simulink model "VehCtrl20260630_18B"  (R2018b)
settings: Solver=FixedStepAuto  StartTime=0.0  StopTime=inf  FixedStep=0.005  RelTol=1e-3
InitFcn:
  | mbd_mpc_consistency_checks(bdroot(gcs));
undefined symbols (not defined in the file): ANG_DEAD, BMS_NormalPwr, BrakeDeadZone, BrkPrsByBrkPct_TB_X, BrkPrsByBrkPct_TB_Y, DELAY_DISCHARGE, DELAY_RCUOFF, DRV_BACKWARD, DRV_BRAKE, DRV_FORWARD, DRV_NEUTRAL, DRV_PARK, DRV_UNPARK, DRV_ZEROTURN, EPB_LOCK, EPB_UNLOCK, ExtraLoadPwr, FanOff, fifo_0_vect, fifo_1_vect, HiFanReq, HV_finished, HV_No_Active, HV_POWER_OFF, HV_POWER_ON, HVDown, HVON, KaTLS_v_DrgUp_X_VehSpd, KeFTM_s_Way1OffDlyTime, KeFTM_TK_Way1CoolLv2OffBatTemp, KeFTM_TK_Way1CoolLv2OffMtrTemp, KeFTM_TK_Way1CoolLv2OnBatTemp, KeFTM_TK_Way1CoolLv2OnMtrTemp, KeFTM_TK_Way1CoolLv3OffBatTemp, KeFTM_TK_Way1CoolLv3OffMtrTemp, KeFTM_TK_Way1CoolLv3OnBatTemp, KeFTM_TK_Way1CoolLv3OnMtrTemp, KeFTM_TK_Way1CoolLv4OffBatTemp, KeFTM_TK_Way1CoolLv4OffMtrTemp, KeFTM_TK_Way1CoolLv4OnBatTemp, KeFTM_TK_Way1CoolLv4OnMtrTemp, Kp1, Kp2, LowFanReq, LQFP, MtrCmdGainFL, MtrCmdGainFR, MtrCmdGainRL, MtrCmdGainRR, MtrPwrFactor_RCU, MtrPwrHighToMidThd, MtrPwrLowToMidThd, MtrPwrMidToHighThd, MtrPwrMidToLowThd, MtrTrqMax, PCT_DEAD, Precharge, PTO_1000, PTO_540, pts1_fifo_0_vect ... (+32)
libraries: mbd_mpc574x_ec_toolbox x175, simulink x110, canmsglib x70
(part 3 of 15)

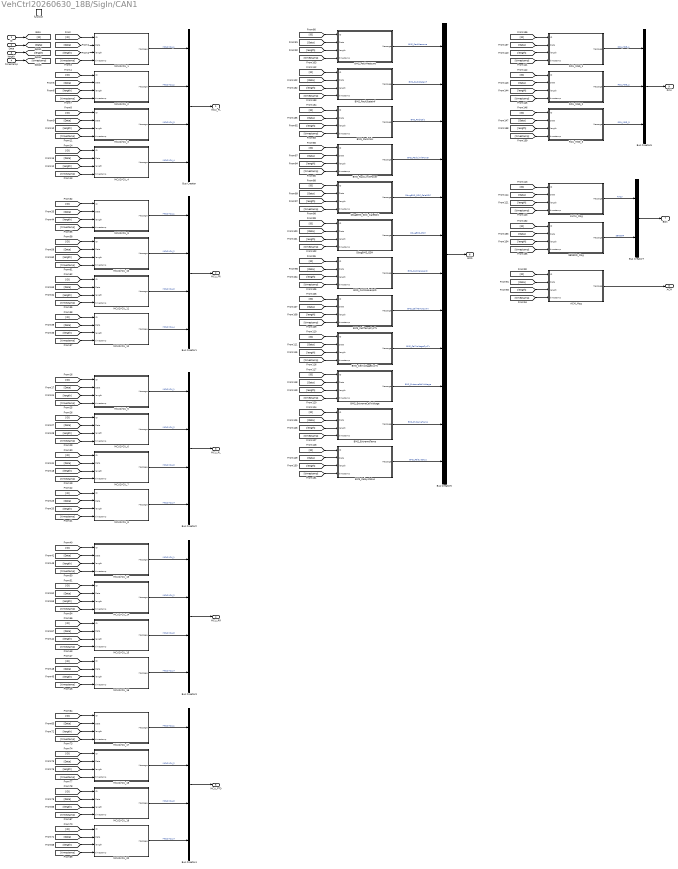
== system VehCtrl20260630_18B/SigIn/CAN1 ==
  ID : Inport
  Data : Inport  Port=2
  length : Inport  Port=3
  timestamp : Inport  Port=4
  function : TriggerPort  TriggerType=function-call  VariantControl=Variant
  ACM_Msg : Subsystem
  AVCU_Msg : Subsystem
  BMS_CANWakeUpID : Subsystem
  BMS_CellTempCycTx : Subsystem
  BMS_CellVoltageCycTx : Subsystem
  BMS_ExtremeCellVoltage : Subsystem
  BMS_ExtremeTemp : Subsystem
  BMS_PackCalc : Subsystem
  BMS_PackLimitPower : Subsystem
  BMS_PackMeasure : Subsystem
  BMS_PackStateInf : Subsystem
  BMS_Relaystatus : Subsystem
  Bus Creator{,1..4} (5 alike) : BusCreator  Inputs=4
  Bus Creator5 : BusCreator  Inputs=12
  Bus Creator6 : BusCreator  Inputs=3
  Bus Creator7 : BusCreator  Inputs=2
  DbugBMS_ESM : Subsystem
  DbugBMS_SOC_CaleSOC : Subsystem
  MCU2VCU_1 : Subsystem
  MCU2VCU_10 : Subsystem
  MCU2VCU_11 : Subsystem
  MCU2VCU_12 : Subsystem
  MCU2VCU_13 : Subsystem
  MCU2VCU_14 : Subsystem
  MCU2VCU_15 : Subsystem
  MCU2VCU_16 : Subsystem
  MCU2VCU_17 : Subsystem
  MCU2VCU_18 : Subsystem
  MCU2VCU_19 : Subsystem
  MCU2VCU_2 : Subsystem
  MCU2VCU_20 : Subsystem
  MCU2VCU_3 : Subsystem
  MCU2VCU_4 : Subsystem
  MCU2VCU_5 : Subsystem
  MCU2VCU_6 : Subsystem
  MCU2VCU_7 : Subsystem
  MCU2VCU_8 : Subsystem
  MCU2VCU_9 : Subsystem
  RCU_MSG_1 : Subsystem
  RCU_MSG_2 : Subsystem
  RCU_MSG_3 : Subsystem
  SENSOR_Msg : Subsystem
  MCU_FL : Outport
  MCU_FR : Outport  Port=2
  MCU_RL : Outport  Port=3
  MCU_RR : Outport  Port=4
  MCU_PTO : Outport  Port=5
  BMS : Outport  Port=6
  BDX : Outport  Port=7
  ACM : Outport  Port=8
  RCU : Outport  Port=9
  wires:
  Bus Creator/1 -> MCU_FL/1
  ID/1 -> [ID]
  Data/1 -> [Data]
  timestamp/1 -> [timestamp]
  length/1 -> [length]
  [ID] -> MCU2VCU_1/1(ID)
  [Data] -> MCU2VCU_1/2(Data)
  [length] -> MCU2VCU_1/3(length)
  [timestamp] -> MCU2VCU_1/4(timestamp)
  [timestamp] -> MCU2VCU_2/4(timestamp)
  [length] -> MCU2VCU_2/3(length)
  [Data] -> MCU2VCU_2/2(Data)
  [ID] -> MCU2VCU_2/1(ID)
  [ID] -> MCU2VCU_3/1(ID)
  [Data] -> MCU2VCU_3/2(Data)
  [length] -> MCU2VCU_3/3(length)
  [timestamp] -> MCU2VCU_3/4(timestamp)
  [timestamp] -> MCU2VCU_4/4(timestamp)
  [length] -> MCU2VCU_4/3(length)
  [Data] -> MCU2VCU_4/2(Data)
  [ID] -> MCU2VCU_4/1(ID)
  MCU2VCU_1/1(Message) -> Bus Creator/1  "MCU2VCU_1"
  MCU2VCU_2/1(Message) -> Bus Creator/2  "MCU2VCU_2"
  MCU2VCU_3/1(Message) -> Bus Creator/3  "MCU2VCU_3"
  MCU2VCU_4/1(Message) -> Bus Creator/4  "MCU2VCU_4"
  MCU2VCU_8/1(Message) -> Bus Creator2/4  "MCU2VCU_4"
  MCU2VCU_7/1(Message) -> Bus Creator2/3  "MCU2VCU_3"
  MCU2VCU_6/1(Message) -> Bus Creator2/2  "MCU2VCU_2"
  MCU2VCU_5/1(Message) -> Bus Creator2/1  "MCU2VCU_1"
  [ID] -> MCU2VCU_8/1(ID)
  [Data] -> MCU2VCU_8/2(Data)
  [length] -> MCU2VCU_8/3(length)
  [timestamp] -> MCU2VCU_8/4(timestamp)
  [timestamp] -> MCU2VCU_7/4(timestamp)
  [length] -> MCU2VCU_7/3(length)
  [Data] -> MCU2VCU_7/2(Data)
  [ID] -> MCU2VCU_7/1(ID)
  [ID] -> MCU2VCU_6/1(ID)
  [Data] -> MCU2VCU_6/2(Data)
  [length] -> MCU2VCU_6/3(length)
  [timestamp] -> MCU2VCU_6/4(timestamp)
  [timestamp] -> MCU2VCU_5/4(timestamp)
  [length] -> MCU2VCU_5/3(length)
  [Data] -> MCU2VCU_5/2(Data)
  [ID] -> MCU2VCU_5/1(ID)
  Bus Creator2/1 -> MCU_RL/1
  Bus Creator3/1 -> MCU_RR/1
  [ID] -> MCU2VCU_13/1(ID)
  [Data] -> MCU2VCU_13/2(Data)
  [length] -> MCU2VCU_13/3(length)
  [timestamp] -> MCU2VCU_13/4(timestamp)
  [timestamp] -> MCU2VCU_14/4(timestamp)
  [length] -> MCU2VCU_14/3(length)
  [Data] -> MCU2VCU_14/2(Data)
  [ID] -> MCU2VCU_14/1(ID)
  [ID] -> MCU2VCU_15/1(ID)
  [Data] -> MCU2VCU_15/2(Data)
  [length] -> MCU2VCU_15/3(length)
  [timestamp] -> MCU2VCU_15/4(timestamp)
  [timestamp] -> MCU2VCU_16/4(timestamp)
  [length] -> MCU2VCU_16/3(length)
  [Data] -> MCU2VCU_16/2(Data)
  [ID] -> MCU2VCU_16/1(ID)
  MCU2VCU_13/1(Message) -> Bus Creator3/1  "MCU2VCU_1"
  MCU2VCU_14/1(Message) -> Bus Creator3/2  "MCU2VCU_2"
  MCU2VCU_15/1(Message) -> Bus Creator3/3  "MCU2VCU_3"
  MCU2VCU_16/1(Message) -> Bus Creator3/4  "MCU2VCU_4"
  MCU2VCU_12/1(Message) -> Bus Creator1/4  "MCU2VCU_4"
  MCU2VCU_11/1(Message) -> Bus Creator1/3  "MCU2VCU_3"
  MCU2VCU_10/1(Message) -> Bus Creator1/2  "MCU2VCU_2"
  MCU2VCU_9/1(Message) -> Bus Creator1/1  "MCU2VCU_1"
  [ID] -> MCU2VCU_12/1(ID)
  [Data] -> MCU2VCU_12/2(Data)
  [length] -> MCU2VCU_12/3(length)
  [timestamp] -> MCU2VCU_12/4(timestamp)
  [timestamp] -> MCU2VCU_11/4(timestamp)
  [length] -> MCU2VCU_11/3(length)
  [Data] -> MCU2VCU_11/2(Data)
  [ID] -> MCU2VCU_11/1(ID)
  [ID] -> MCU2VCU_10/1(ID)
  [Data] -> MCU2VCU_10/2(Data)
  [length] -> MCU2VCU_10/3(length)
  [timestamp] -> MCU2VCU_10/4(timestamp)
  [timestamp] -> MCU2VCU_9/4(timestamp)
  [length] -> MCU2VCU_9/3(length)
  [Data] -> MCU2VCU_9/2(Data)
  [ID] -> MCU2VCU_9/1(ID)
  Bus Creator1/1 -> MCU_FR/1
  MCU2VCU_20/1(Message) -> Bus Creator4/4  "MCU2VCU_4"
  MCU2VCU_19/1(Message) -> Bus Creator4/3  "MCU2VCU_3"
  MCU2VCU_18/1(Message) -> Bus Creator4/2  "MCU2VCU_2"
  MCU2VCU_17/1(Message) -> Bus Creator4/1  "MCU2VCU_1"
  [ID] -> MCU2VCU_20/1(ID)
  [Data] -> MCU2VCU_20/2(Data)
  [length] -> MCU2VCU_20/3(length)
  [timestamp] -> MCU2VCU_20/4(timestamp)
  [timestamp] -> MCU2VCU_19/4(timestamp)
  [length] -> MCU2VCU_19/3(length)
  [Data] -> MCU2VCU_19/2(Data)
  [ID] -> MCU2VCU_19/1(ID)
  [ID] -> MCU2VCU_18/1(ID)
  [Data] -> MCU2VCU_18/2(Data)
  [length] -> MCU2VCU_18/3(length)
  [timestamp] -> MCU2VCU_18/4(timestamp)
  [timestamp] -> MCU2VCU_17/4(timestamp)
  [length] -> MCU2VCU_17/3(length)
  [Data] -> MCU2VCU_17/2(Data)
  [ID] -> MCU2VCU_17/1(ID)
  Bus Creator4/1 -> MCU_PTO/1
  [timestamp] -> BMS_CellTempCycTx/4(timestamp)
  [timestamp] -> ACM_Msg/4(timestamp)
  [ID] -> BMS_Relaystatus/1(ID)
  BMS_ExtremeCellVoltage/1(Message) -> Bus Creator5/10  "BMS_ExtremeCellVoltage"
  [Data] -> DbugBMS_ESM/2(Data)
  BMS_CellTempCycTx/1(Message) -> Bus Creator5/8  "BMS_CellTempCycTx"
  BMS_CellVoltageCycTx/1(Message) -> Bus Creator5/9  "BMS_CellVoltageCycTx"
  [ID] -> AVCU_Msg/1(ID)
  [length] -> BMS_Relaystatus/3(length)
  [timestamp] -> BMS_CANWakeUpID/4(timestamp)
  [length] -> BMS_CellTempCycTx/3(length)
  DbugBMS_SOC_CaleSOC/1(Message) -> Bus Creator5/5  "DbugBMS_SOC_CaleSOC"
  [timestamp] -> BMS_Relaystatus/4(timestamp)
  [timestamp] -> BMS_PackStateInf/4(timestamp)
  [ID] -> BMS_ExtremeCellVoltage/1(ID)
  BMS_Relaystatus/1(Message) -> Bus Creator5/12  "BMS_Relaystatus"
  [Data] -> BMS_CANWakeUpID/2(Data)
  [length] -> BMS_ExtremeCellVoltage/3(length)
  [timestamp] -> BMS_ExtremeCellVoltage/4(timestamp)
  [Data] -> BMS_PackLimitPower/2(Data)
  [Data] -> BMS_ExtremeCellVoltage/2(Data)
  [Data] -> BMS_PackStateInf/2(Data)
  [Data] -> BMS_ExtremeTemp/2(Data)
  DbugBMS_ESM/1(Message) -> Bus Creator5/6  "DbugBMS_ESM"
  [timestamp] -> BMS_PackCalc/4(timestamp)
  [ID] -> BMS_CANWakeUpID/1(ID)
  [Data] -> BMS_CellTempCycTx/2(Data)
  [length] -> AVCU_Msg/3(length)
  [length] -> BMS_PackCalc/3(length)
  [ID] -> ACM_Msg/1(ID)
  [timestamp] -> BMS_CellVoltageCycTx/4(timestamp)
  ACM_Msg/1(Message) -> ACM/1
  Bus Creator5/1 -> BMS/1
  [length] -> ACM_Msg/3(length)
  [Data] -> BMS_PackMeasure/2(Data)
  [timestamp] -> BMS_PackLimitPower/4(timestamp)
  [Data] -> BMS_CellVoltageCycTx/2(Data)
  [ID] -> BMS_PackLimitPower/1(ID)
  [Data] -> DbugBMS_SOC_CaleSOC/2(Data)
  BMS_CANWakeUpID/1(Message) -> Bus Creator5/7  "BMS_CANWakeUpID"
  [ID] -> BMS_PackCalc/1(ID)
  [length] -> BMS_PackMeasure/3(length)
  BMS_PackMeasure/1(Message) -> Bus Creator5/1  "BMS_PackMeasure"
  [Data] -> BMS_Relaystatus/2(Data)
  [Data] -> BMS_PackCalc/2(Data)
  [length] -> BMS_PackLimitPower/3(length)
  [ID] -> BMS_ExtremeTemp/1(ID)
  BMS_PackCalc/1(Message) -> Bus Creator5/3  "BMS_PackCalc"
  [timestamp] -> BMS_ExtremeTemp/4(timestamp)
  BMS_PackStateInf/1(Message) -> Bus Creator5/2  "BMS_PackStateInf"
  [length] -> BMS_CellVoltageCycTx/3(length)
  [timestamp] -> DbugBMS_ESM/4(timestamp)
  [ID] -> BMS_CellVoltageCycTx/1(ID)
  [length] -> BMS_CANWakeUpID/3(length)
  [length] -> DbugBMS_ESM/3(length)
  BMS_PackLimitPower/1(Message) -> Bus Creator5/4  "BMS_PackLimitPower"
  [ID] -> DbugBMS_SOC_CaleSOC/1(ID)
  [length] -> BMS_ExtremeTemp/3(length)
  [timestamp] -> DbugBMS_SOC_CaleSOC/4(timestamp)
  [ID] -> BMS_PackStateInf/1(ID)
  [Data] -> ACM_Msg/2(Data)
  [ID] -> BMS_CellTempCycTx/1(ID)
  [Data] -> AVCU_Msg/2(Data)
  [ID] -> BMS_PackMeasure/1(ID)
  [timestamp] -> BMS_PackMeasure/4(timestamp)
  BMS_ExtremeTemp/1(Message) -> Bus Creator5/11  "BMS_ExtremeTemp"
  [ID] -> DbugBMS_ESM/1(ID)
  [length] -> BMS_PackStateInf/3(length)
  [timestamp] -> AVCU_Msg/4(timestamp)
  [length] -> DbugBMS_SOC_CaleSOC/3(length)
  RCU_MSG_2/1(Message) -> Bus Creator6/2  "RCU_MSG_2"
  [length] -> RCU_MSG_3/3(length)
  RCU_MSG_3/1(Message) -> Bus Creator6/3  "RCU_MSG_3"
  [Data] -> RCU_MSG_2/2(Data)
  [length] -> RCU_MSG_2/3(length)
  [Data] -> RCU_MSG_1/2(Data)
  [Data] -> RCU_MSG_3/2(Data)
  [ID] -> RCU_MSG_2/1(ID)
  [timestamp] -> RCU_MSG_2/4(timestamp)
  [ID] -> RCU_MSG_3/1(ID)
  RCU_MSG_1/1(Message) -> Bus Creator6/1  "RCU_MSG_1"
  [length] -> RCU_MSG_1/3(length)
  [ID] -> RCU_MSG_1/1(ID)
  [timestamp] -> RCU_MSG_3/4(timestamp)
  Bus Creator6/1 -> RCU/1
  [timestamp] -> RCU_MSG_1/4(timestamp)
  [ID] -> SENSOR_Msg/1(ID)
  [Data] -> SENSOR_Msg/2(Data)
  [length] -> SENSOR_Msg/3(length)
  [timestamp] -> SENSOR_Msg/4(timestamp)
  SENSOR_Msg/1(Message) -> Bus Creator7/2  "SENSOR"
  AVCU_Msg/1(Message) -> Bus Creator7/1  "AVCU"
  Bus Creator7/1 -> BDX/1

== system VehCtrl20260630_18B/SigIn/DI ==
  note: DI PULLDOWN
  note: DI PULLUP
  Bus Creator : BusCreator  Inputs=14
  DI01 : mbd_mpc574x_ec_toolbox/GPIO Blocks/Digital_Input  gpio_pin=PTG5: [SIUL2_GPIO101 | General Purpose IO PG[5]]  pull_resistor=None
  DI02 : mbd_mpc574x_ec_toolbox/GPIO Blocks/Digital_Input  gpio_pin=PTG9: [SIUL2_GPIO105 | General Purpose IO PG[9]]  pull_resistor=None
  DI03 : mbd_mpc574x_ec_toolbox/GPIO Blocks/Digital_Input  gpio_pin=PTC11: [SIUL2_GPIO43 | General Purpose IO PC[11]]  pull_resistor=None
  DI04 : mbd_mpc574x_ec_toolbox/GPIO Blocks/Digital_Input  gpio_pin=PTA9: [SIUL2_GPIO9 | General Purpose IO PA[9]]  pull_resistor=None
  DI07 : mbd_mpc574x_ec_toolbox/GPIO Blocks/Digital_Input  gpio_pin=PTA0: [SIUL2_GPIO0 | General Purpose IO PA[0]]  pull_resistor=None
  DI08 : mbd_mpc574x_ec_toolbox/GPIO Blocks/Digital_Input  gpio_pin=PTD11: [SIUL2_GPIO59 | General Purpose IO PD[11]]  pull_resistor=None
  DI09 : mbd_mpc574x_ec_toolbox/GPIO Blocks/Digital_Input  gpio_pin=PTG6: [SIUL2_GPIO102 | General Purpose IO PG[6]]  pull_resistor=None
  DI10 : mbd_mpc574x_ec_toolbox/GPIO Blocks/Digital_Input  gpio_pin=PTG2: [SIUL2_GPIO98 | General Purpose IO PG[2]]  pull_resistor=None
  DI12 : mbd_mpc574x_ec_toolbox/GPIO Blocks/Digital_Input  gpio_pin=PTF13: [SIUL2_GPIO93 | General Purpose IO PF[13]]  pull_resistor=None
  DI13 : mbd_mpc574x_ec_toolbox/GPIO Blocks/Digital_Input  gpio_pin=PTG4: [SIUL2_GPIO100 | General Purpose IO PG[4]]  pull_resistor=None
  DI15 : mbd_mpc574x_ec_toolbox/GPIO Blocks/Digital_Input  gpio_pin=PTF12: [SIUL2_GPIO92 | General Purpose IO PF[12]]  pull_resistor=None
  DI16 : mbd_mpc574x_ec_toolbox/GPIO Blocks/Digital_Input  gpio_pin=PTG7: [SIUL2_GPIO103 | General Purpose IO PG[7]]  pull_resistor=None
  DI17 : mbd_mpc574x_ec_toolbox/GPIO Blocks/Digital_Input  gpio_pin=PTD10: [SIUL2_GPIO58 | General Purpose IO PD[10]]  pull_resistor=None
  DI18 : mbd_mpc574x_ec_toolbox/GPIO Blocks/Digital_Input  gpio_pin=PTG10: [SIUL2_GPIO106 | General Purpose IO PG[10]]  pull_resistor=None
  DI_31_32_33_34 : Subsystem  Commented=on
  Data Store Read : DataStoreRead  DataStoreName=DI07
  Data Store Read1 : DataStoreRead  DataStoreName=DI10
  Data Store Read10 : DataStoreRead  DataStoreName=DI04
  Data Store Read11 : DataStoreRead  DataStoreName=DI12
  Data Store Read12 : DataStoreRead  DataStoreName=DI08
  Data Store Read13 : DataStoreRead  DataStoreName=DI09
  Data Store Read2 : DataStoreRead  DataStoreName=DI13
  Data Store Read3 : DataStoreRead  DataStoreName=DI15
  Data Store Read4 : DataStoreRead  DataStoreName=DI16
  Data Store Read5 : DataStoreRead  DataStoreName=DI17
  Data Store Read6 : DataStoreRead  DataStoreName=DI18
  Data Store Read7 : DataStoreRead  DataStoreName=DI01
  Data Store Read8 : DataStoreRead  DataStoreName=DI02
  Data Store Read9 : DataStoreRead  DataStoreName=DI03
  Data Store Write : DataStoreWrite  DataStoreName=DI07
  Data Store Write1 : DataStoreWrite  DataStoreName=DI01
  Data Store Write10 : DataStoreWrite  DataStoreName=DI04
  Data Store Write11 : DataStoreWrite  DataStoreName=DI12
  Data Store Write12 : DataStoreWrite  DataStoreName=DI08
  Data Store Write13 : DataStoreWrite  DataStoreName=DI09
  Data Store Write2 : DataStoreWrite  DataStoreName=DI10
  Data Store Write3 : DataStoreWrite  DataStoreName=DI13
  Data Store Write4 : DataStoreWrite  DataStoreName=DI15
  Data Store Write5 : DataStoreWrite  DataStoreName=DI16
  Data Store Write6 : DataStoreWrite  DataStoreName=DI17
  Data Store Write7 : DataStoreWrite  DataStoreName=DI18
  Data Store Write8 : DataStoreWrite  DataStoreName=DI02
  Data Store Write9 : DataStoreWrite  DataStoreName=DI03
  DI : Outport
  wires:
  DI07/1 -> Data Store Write/1
  DI01/1 -> Data Store Write1/1
  DI10/1 -> Data Store Write2/1
  DI13/1 -> Data Store Write3/1
  DI15/1 -> Data Store Write4/1
  DI17/1 -> Data Store Write6/1
  DI16/1 -> Data Store Write5/1
  DI18/1 -> Data Store Write7/1
  DI09/1 -> Data Store Write13/1
  DI08/1 -> Data Store Write12/1
  DI12/1 -> Data Store Write11/1
  DI04/1 -> Data Store Write10/1
  DI02/1 -> Data Store Write8/1
  DI03/1 -> Data Store Write9/1
  Data Store Read/1 -> Bus Creator/1  "DI07"
  Data Store Read1/1 -> Bus Creator/2  "DI10"
  Data Store Read2/1 -> Bus Creator/3  "DI13"
  Data Store Read3/1 -> Bus Creator/4  "DI15"
  Data Store Read4/1 -> Bus Creator/5  "DI16"
  Data Store Read5/1 -> Bus Creator/6  "DI17"
  Data Store Read6/1 -> Bus Creator/7  "DI18"
  Data Store Read7/1 -> Bus Creator/8  "DI01"
  Data Store Read8/1 -> Bus Creator/9  "DI02"
  Data Store Read9/1 -> Bus Creator/10  "DI03"
  Data Store Read10/1 -> Bus Creator/11  "DI04"
  Data Store Read11/1 -> Bus Creator/12  "DI12"
  Data Store Read12/1 -> Bus Creator/13  "DI08"
  Data Store Read13/1 -> Bus Creator/14  "DI09"
  Bus Creator/1 -> DI/1

== system VehCtrl20260630_18B/SigIn/PWM ==
  note: DI PWM PULLDOWN
  note: DI PWM PULLUP
  Bus Creator : BusCreator  Inputs=8
  Data Store Read : DataStoreRead  DataStoreName=DI31_PWM_DC
  Data Store Read1 : DataStoreRead  DataStoreName=DI31_PWM_FRQ
  Data Store Read2 : DataStoreRead  DataStoreName=DI32_PWM_DC
  Data Store Read3 : DataStoreRead  DataStoreName=DI32_PWM_FRQ
  Data Store Read4 : DataStoreRead  DataStoreName=DI33_PWM_DC
  Data Store Read5 : DataStoreRead  DataStoreName=DI33_PWM_FRQ
  Data Store Read6 : DataStoreRead  DataStoreName=DI34_PWM_DC
  Data Store Read7 : DataStoreRead  DataStoreName=DI34_PWM_FRQ
  Data Store Write : DataStoreWrite  DataStoreName=DI31_PWM_DC
  Data Store Write1 : DataStoreWrite  DataStoreName=DI31_PWM_FRQ
  Data Store Write2 : DataStoreWrite  DataStoreName=DI32_PWM_DC
  Data Store Write3 : DataStoreWrite  DataStoreName=DI32_PWM_FRQ
  Data Store Write4 : DataStoreWrite  DataStoreName=DI33_PWM_DC
  Data Store Write5 : DataStoreWrite  DataStoreName=DI33_PWM_FRQ
  Data Store Write6 : DataStoreWrite  DataStoreName=DI34_PWM_FRQ
  Data Store Write7 : DataStoreWrite  DataStoreName=DI34_PWM_DC
  PWM_PTS1 : Subsystem
  PWM_PTS2 : Subsystem
  PWM_PTS3 : Subsystem
  PWM_PTS4 : Subsystem
  Subsystem : Subsystem  Commented=on
  eTimer_Arm_Capture : mbd_mpc574x_ec_toolbox/Motor Control Blocks/eTIMER Blocks/eTimer_Arm_Capture  etimerModule=0  etimerChannel=2  etimerArmAction=Start
  eTimer_Arm_Capture1 : mbd_mpc574x_ec_toolbox/Motor Control Blocks/eTIMER Blocks/eTimer_Arm_Capture  etimerModule=1  etimerChannel=2  etimerArmAction=Start
  eTimer_Arm_Capture2 : mbd_mpc574x_ec_toolbox/Motor Control Blocks/eTIMER Blocks/eTimer_Arm_Capture  etimerModule=1  etimerChannel=1  etimerArmAction=Start
  eTimer_Arm_Capture3 : mbd_mpc574x_ec_toolbox/Motor Control Blocks/eTIMER Blocks/eTimer_Arm_Capture  etimerModule=1  etimerChannel=3  etimerArmAction=Start
  PWMIn : Outport
  wires:
  Bus Creator/1 -> PWMIn/1
  Data Store Read7/1 -> Bus Creator/8  "DI34_PWM_FRQ"
  Data Store Read6/1 -> Bus Creator/7  "DI34_PWM_DC"
  Data Store Read5/1 -> Bus Creator/6  "DI33_PWM_FRQ"
  Data Store Read4/1 -> Bus Creator/5  "DI33_PWM_DC"
  Data Store Read3/1 -> Bus Creator/4  "DI32_PWM_FRQ"
  Data Store Read2/1 -> Bus Creator/3  "DI32_PWM_DC"
  Data Store Read1/1 -> Bus Creator/2  "DI31_PWM_FRQ"
  Data Store Read/1 -> Bus Creator/1  "DI31_PWM_DC"
  PWM_PTS4/1(DC) -> Data Store Write/1
  PWM_PTS4/2(freq) -> Data Store Write1/1
  PWM_PTS1/1(DC) -> Data Store Write2/1
  PWM_PTS1/2(freq) -> Data Store Write3/1
  PWM_PTS2/1(DC) -> Data Store Write4/1
  PWM_PTS2/2(freq) -> Data Store Write5/1
  PWM_PTS3/2(freq) -> Data Store Write6/1
  PWM_PTS3/1(DC) -> Data Store Write7/1

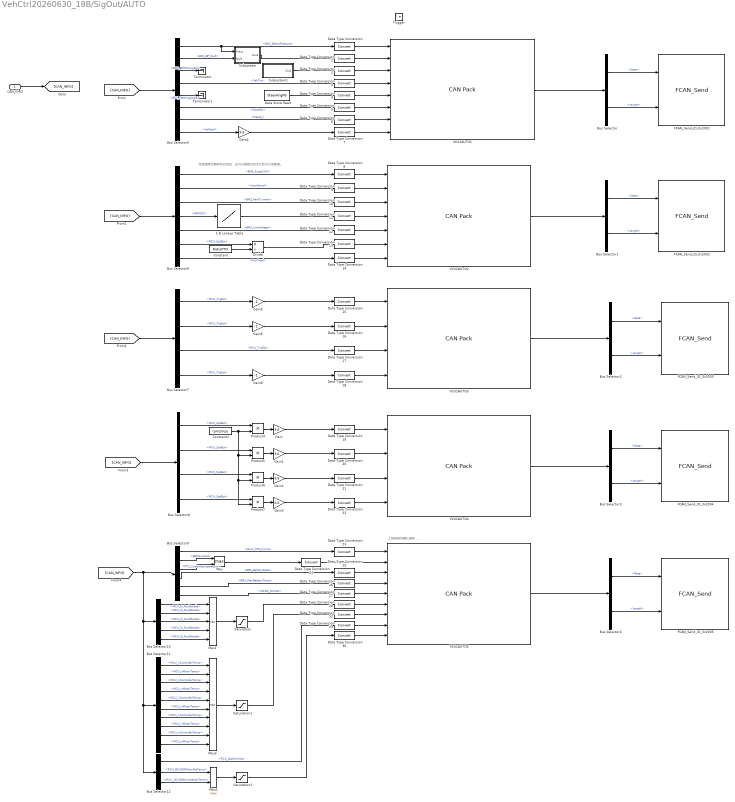
== system VehCtrl20260630_18B/SigOut/AUTO ==
  note: 上报信息待确认更新……
  note: 当前使用的是BMS的低压，也可以替换为DCDC或VCU采集值。
  "CAN_INFO " : Inport
  Trigger : TriggerPort  VariantControl=Variant  PortDimensions=1
  1-D Lookup Table : Lookup_n-D  NumberOfTableDimensions=1  BreakpointsForDimension1=SOC_display_x  Table=SOC_display_y  InternalRulePriority=Speed  RndMeth=Simplest  InputSameDT=on
  Bus Selector{,1..4} (5 alike) : BusSelector  OutputSignals=Data,Length
  Bus Selector10 : BusSelector  OutputSignals=MCU_FL.MCU2VCU_3.MCU_N_FaultGrade,MCU_FR.MCU2VCU_3.MCU_N_FaultGrade,MCU_RL.MCU2VCU_3.MCU_N_FaultGrade,MCU_RR.MCU2VCU_3.MCU_N_FaultGrade,MCU_PTO.MCU2VCU_3.MCU_N_FaultGrade
  Bus Selector11 : BusSelector  OutputSignals=MCU_FL.MCU2VCU_2.MCU_nControllerTemp,MCU_FL.MCU2VCU_2.MCU_nMotorTemp,MCU_FR.MCU2VCU_2.MCU_nControllerTemp,MCU_FR.MCU2VCU_2.MCU_nMotorTemp,MCU_RL.MCU2VCU_2.MCU_nControllerTemp,MCU_RL.MCU2VCU_2.MCU_nMotorTemp,MCU_RR.MCU2VCU_2.MCU_nControllerTemp,MCU_RR.MCU2VCU_2.MCU_nMotorTemp,MCU_PTO.MCU2VCU_2.MCU_nControllerTemp,MCU_PTO.MCU2VCU_2.MCU_nMotorTemp
  Bus Selector12 : BusSelector  OutputSignals=RCU.RCU_MSG_1.RCU_ActWorkSts,RCU.RCU_MSG_3.RCU_GCUISGMotorActTemp,RCU.RCU_MSG_3.RCU_GCUISGInverterActTemp
  Bus Selector5 : BusSelector  OutputSignals=BDX.AVCU.BDX_BrakePressure,BDX.AVCU.BDX_BP_fault,BMS.DbugBMS_ESM.ESM_BMSChargSts,VehTrq,BDX.AVCU.BDX_SteeringAngle,CMD.ModeStr,Ready,VehSpd
  Bus Selector6 : BusSelector  OutputSignals=BMS.BMS_PackCalc.BMS_SupplyVol,DAQ.LiqudLevel,BMS.BMS_PackMeasure.BMS_PackCurrent,BMS.DbugBMS_SOC_CaleSOC.APPSOC,BMS.BMS_PackMeasure.BMS_LineVoltage,MCU_PTO.MCU2VCU_1.MCU_SpdEst,PwrTotal
  Bus Selector7 : BusSelector  OutputSignals=MCU_FL.MCU2VCU_1.MCU_TrqEst,MCU_FR.MCU2VCU_1.MCU_TrqEst,MCU_RL.MCU2VCU_1.MCU_TrqEst,MCU_RR.MCU2VCU_1.MCU_TrqEst
  Bus Selector8 : BusSelector  OutputSignals=MCU_FL.MCU2VCU_1.MCU_SpdEst,MCU_FR.MCU2VCU_1.MCU_SpdEst,MCU_RL.MCU2VCU_1.MCU_SpdEst,MCU_RR.MCU2VCU_1.MCU_SpdEst
  Bus Selector9 : BusSelector  OutputSignals=ACM.Work_STS_Comp,DAQ.BatTempOut,PTC.signal1.PTC_Coolanttemperature,BMS.BMS_PackStateInf.BMS_BatteryState,BMS.BMS_ExtremeTemp.BMS_MaxBatteryTemp,DCDC.DCDC_WrkSts
  Constant : Constant  Value=RatioPTO
  Constant2 : Constant  Value=rpm2mps
  Data Store Read : DataStoreRead  DataStoreName=SteerAngFB
  Data Type Conversion{,1..31} (32 alike) : DataTypeConversion
  Divide : Product  Inputs=*/
  FCAN_Send_ID_0x2001 : mbd_mpc574x_ec_toolbox/Communication Blocks/CAN Blocks/FCAN_Send  Priority=2  can_instance=1  can_mode=Non-blocking  can_timeout_ms=0  can_mb_idx=46  can_extended_id=on  can_is_remote=off  can_id=2001  show_adv_opts=off  can_fd_enable=off  can_enable_brs=off  can_fd_padding=0
      settings: SourceProductName=NXP Model-Based Design Toolbox for MPC57xx MCUs
  FCAN_Send_ID_0x2002 : mbd_mpc574x_ec_toolbox/Communication Blocks/CAN Blocks/FCAN_Send  Priority=2  can_instance=1  can_mode=Non-blocking  can_timeout_ms=0  can_mb_idx=40  can_extended_id=on  can_is_remote=off  can_id=2002  show_adv_opts=off  can_fd_enable=off  can_enable_brs=off  can_fd_padding=0
      settings: SourceProductName=NXP Model-Based Design Toolbox for MPC57xx MCUs
  FCAN_Send_ID_0x2003 : mbd_mpc574x_ec_toolbox/Communication Blocks/CAN Blocks/FCAN_Send  Priority=2  can_instance=1  can_mode=Non-blocking  can_timeout_ms=0  can_mb_idx=41  can_extended_id=on  can_is_remote=off  can_id=2003  show_adv_opts=off  can_fd_enable=off  can_enable_brs=off  can_fd_padding=0
      settings: SourceProductName=NXP Model-Based Design Toolbox for MPC57xx MCUs
  FCAN_Send_ID_0x2004 : mbd_mpc574x_ec_toolbox/Communication Blocks/CAN Blocks/FCAN_Send  Priority=2  can_instance=1  can_mode=Non-blocking  can_timeout_ms=0  can_mb_idx=42  can_extended_id=on  can_is_remote=off  can_id=2004  show_adv_opts=off  can_fd_enable=off  can_enable_brs=off  can_fd_padding=0
      settings: SourceProductName=NXP Model-Based Design Toolbox for MPC57xx MCUs
  FCAN_Send_ID_0x2005 : mbd_mpc574x_ec_toolbox/Communication Blocks/CAN Blocks/FCAN_Send  Priority=2  can_instance=1  can_mode=Non-blocking  can_timeout_ms=0  can_mb_idx=39  can_extended_id=on  can_is_remote=off  can_id=2005  show_adv_opts=off  can_fd_enable=off  can_enable_brs=off  can_fd_padding=0
      settings: SourceProductName=NXP Model-Based Design Toolbox for MPC57xx MCUs
  Gain{,1..4} (5 alike) : Gain  Gain=3.6
  Gain5 : Gain  Gain=-1
  Gain6 : Gain  Gain=-1
  Gain8 : Gain  Gain=-1
  Max : MinMax  Function=max  Inputs=2
  Max1 : MinMax  Function=max  Inputs=5
  Max2 : MinMax  Function=max  Inputs=2
  Max3 : MinMax  Function=max  Inputs=10
  Product{4..7} (4 alike) : Product
  Saturation : Saturate  UpperLimit=3  LowerLimit=0
  Saturation1 : Saturate  UpperLimit=200  LowerLimit=-50
  Saturation2 : Saturate  UpperLimit=200  LowerLimit=-50
  Subsystem : Subsystem
  Subsystem1 : Subsystem
  Terminator : Terminator
  Terminator1 : Terminator
  VCU2AUTO1 : canmsglib/CAN Pack  CANdbFile=D:\VCU\VCU_AgriculturalMachinery_ChangChun\VCU_AgriculturalMachinery_260519_ChangChun\CAN协议0519\AUTO\TractorAuto_dbc_WhlTrq_0p1.dbc  MsgList=VCU2AUTO1  MsgName=VCU2AUTO1  MsgIDType=Extended (29-bit identifier)  MsgIdentifier=8193  MsgLength=8  SignalInfo=VCU_BrkPrs$48$8$1$2$1$0$1$0$0$200$#VCU_BrkSt$60$2$1$2$1$0$1$0$0$3$#VCU_CtrMode$62$2$1$2$1$0$1$0$0$3$#VCU_DrvTrqTotal$16$16$1$2$1$0$1$-30000$-30000$30000$#VCU_StrAng$32$16$1$2$1$0$1.000000e-02$-100$-100$100$#VCU_StrSt$58$2$1$2$1$0$1$0$0$3$#VCU_VcuSt$56$2$1$2$1$0$1$0$0$3$#VCU_VehSpd$0$16$1$2$1$0$1.000000e-02$-20$-20$40$#  NSignals=8  StartBits=str2num('[int32(48);int32(60);int32(62);int32(16);int32(32);int32(58);int32(56);int32(0)]')  SignalSizes=str2num('[int32(8);int32(2);int32(2);int32(16);int32(16);int32(2);int32(2);int32(16)]')  ByteOrders=str2num('[int32(1);int32(1);int32(1);int32(1);int32(1);int32(1);int32(1);int32(1)]')  DataTypes=str2num('[int32(2);int32(2);int32(2);int32(2);int32(2);int32(2);int32(2);int32(2)]')  MultiplexTypes=str2num('[int32(1);int32(1);int32(1);int32(1);int32(1);int32(1);int32(1);int32(1)]')  MultiplexValues=str2num('[double(0);double(0);double(0);double(0);double(0);double(0);double(0);double(0)]')  Factors=str2num('[double(1);double(1);double(1);double(1);double(1.000000e-02);double(1);double(1);double(1.000000e-02)]')  Offsets=str2num('[double(0);double(0);double(0);double(-30000);double(-100);double(0);double(0);double(-20)]')  Minimums=str2num('[double(0);double(0);double(0);double(-30000);double(-100);double(0);double(0);double(-20)]')  Maximums=str2num('[double(200);double(3);double(3);double(30000);double(100);double(3);double(3);double(40)]')  Remote=off  ApplyMinMax=off  BusOutput=on
      settings: SourceProductName=Simulink Real-Time  SourceProductBaseCode=XP  DataFormat=CANdb specified signals
  VCU2AUTO2 : canmsglib/CAN Pack  CANdbFile=E:\硕士工作\0.本周工作\20260428_changchun\VCU_AgriculturalMachinery_260428_ChangChun\VCU_AgriculturalMachinery_260428_ChangChun\CAN协议9.1\AUTO\TractorAuto_Intel.dbc  MsgList=VCU2AUTO2  MsgName=VCU2AUTO2  MsgIDType=Extended (29-bit identifier)  MsgIdentifier=8194  MsgLength=8  SignalInfo=VCU_BatVol$56$8$1$2$1$0$2.000000e-01$0$0$50$#VCU_Fuel$48$8$1$2$1$0$1$0$0$100$#VCU_HvCur$24$8$1$2$1$0$2$-100$-100$400$#VCU_HvSoc$40$8$1$2$1$0$1$0$0$100$#VCU_HvVol$16$8$1$2$1$0$2$0$0$500$#VCU_PtoSpd$0$16$1$2$1$0$1.000000e-01$-3000$-3000$3000$#VCU_PwrTotal$32$8$1$2$1$0$1$-50$-50$200$#  NSignals=7  StartBits=str2num('[int32(56);int32(48);int32(24);int32(40);int32(16);int32(0);int32(32)]')  SignalSizes=str2num('[int32(8);int32(8);int32(8);int32(8);int32(8);int32(16);int32(8)]')  ByteOrders=str2num('[int32(1);int32(1);int32(1);int32(1);int32(1);int32(1);int32(1)]')  DataTypes=str2num('[int32(2);int32(2);int32(2);int32(2);int32(2);int32(2);int32(2)]')  MultiplexTypes=str2num('[int32(1);int32(1);int32(1);int32(1);int32(1);int32(1);int32(1)]')  MultiplexValues=str2num('[double(0);double(0);double(0);double(0);double(0);double(0);double(0)]')  Factors=str2num('[double(2.000000e-01);double(1);double(2);double(1);double(2);double(1.000000e-01);double(1)]')  Offsets=str2num('[double(0);double(0);double(-100);double(0);double(0);double(-3000);double(-50)]')  Minimums=str2num('[double(0);double(0);double(-100);double(0);double(0);double(-3000);double(-50)]')  Maximums=str2num('[double(50);double(100);double(400);double(100);double(500);double(3000);double(200)]')  Remote=off  ApplyMinMax=off  BusOutput=on
      settings: SourceProductName=Simulink Real-Time  SourceProductBaseCode=XP  DataFormat=CANdb specified signals
  VCU2AUTO3 : canmsglib/CAN Pack  CANdbFile=D:\VCU\VCU_AgriculturalMachinery_ChangChun\VCU_AgriculturalMachinery_260519_ChangChun\CAN协议0519\AUTO\TractorAuto_dbc_WhlTrq_0p1.dbc  MsgList=VCU2AUTO3  MsgName=VCU2AUTO3  MsgIDType=Extended (29-bit identifier)  MsgIdentifier=8195  MsgLength=8  SignalInfo=VCU_WhlTrqFL$0$16$1$2$1$0$1.000000e-01$-3000$-3000$3000$#VCU_WhlTrqFR$16$16$1$2$1$0$1.000000e-01$-3000$-3000$3000$#VCU_WhlTrqRL$32$16$1$2$1$0$1.000000e-01$-3000$-3000$3000$#VCU_WhlTrqRR$48$16$1$2$1$0$1.000000e-01$-3000$-3000$3000$#  NSignals=4  StartBits=str2num('[int32(0);int32(16);int32(32);int32(48)]')  SignalSizes=str2num('[int32(16);int32(16);int32(16);int32(16)]')  ByteOrders=str2num('[int32(1);int32(1);int32(1);int32(1)]')  DataTypes=str2num('[int32(2);int32(2);int32(2);int32(2)]')  MultiplexTypes=str2num('[int32(1);int32(1);int32(1);int32(1)]')  MultiplexValues=str2num('[double(0);double(0);double(0);double(0)]')  Factors=str2num('[double(1.000000e-01);double(1.000000e-01);double(1.000000e-01);double(1.000000e-01)]')  Offsets=str2num('[double(-3000);double(-3000);double(-3000);double(-3000)]')  Minimums=str2num('[double(-3000);double(-3000);double(-3000);double(-3000)]')  Maximums=str2num('[double(3000);double(3000);double(3000);double(3000)]')  Remote=off  ApplyMinMax=off  BusOutput=on
      settings: SourceProductName=Simulink Real-Time  SourceProductBaseCode=XP  DataFormat=CANdb specified signals
  VCU2AUTO4 : canmsglib/CAN Pack  CANdbFile=E:\硕士工作\0.本周工作\20260428_changchun\VCU_AgriculturalMachinery_260428_ChangChun\VCU_AgriculturalMachinery_260428_ChangChun\CAN协议9.1\AUTO\TractorAuto_Intel.dbc  MsgList=VCU2AUTO4  MsgName=VCU2AUTO4  MsgIDType=Extended (29-bit identifier)  MsgIdentifier=8196  MsgLength=8  SignalInfo=VCU_WhlSpdFL$0$16$1$2$1$0$1.000000e-02$-20$-20$40$#VCU_WhlSpdFR$16$16$1$2$1$0$1.000000e-02$-20$-20$40$#VCU_WhlSpdRL$32$16$1$2$1$0$1.000000e-02$-20$-20$40$#VCU_WhlSpdRR$48$16$1$2$1$0$1.000000e-02$-20$-20$40$#  NSignals=4  StartBits=str2num('[int32(0);int32(16);int32(32);int32(48)]')  SignalSizes=str2num('[int32(16);int32(16);int32(16);int32(16)]')  ByteOrders=str2num('[int32(1);int32(1);int32(1);int32(1)]')  DataTypes=str2num('[int32(2);int32(2);int32(2);int32(2)]')  MultiplexTypes=str2num('[int32(1);int32(1);int32(1);int32(1)]')  MultiplexValues=str2num('[double(0);double(0);double(0);double(0)]')  Factors=str2num('[double(1.000000e-02);double(1.000000e-02);double(1.000000e-02);double(1.000000e-02)]')  Offsets=str2num('[double(-20);double(-20);double(-20);double(-20)]')  Minimums=str2num('[double(-20);double(-20);double(-20);double(-20)]')  Maximums=str2num('[double(40);double(40);double(40);double(40)]')  Remote=off  ApplyMinMax=off  BusOutput=on
      settings: SourceProductName=Simulink Real-Time  SourceProductBaseCode=XP  DataFormat=CANdb specified signals
  VCU2AUTO5 : canmsglib/CAN Pack  CANdbFile=E:\硕士工作\0.本周工作\20260428_changchun\VCU_AgriculturalMachinery_260428_ChangChun\VCU_AgriculturalMachinery_260428_ChangChun\CAN协议9.1\AUTO\TractorAuto_Intel.dbc  MsgList=VCU2AUTO5  MsgName=VCU2AUTO5  MsgIDType=Extended (29-bit identifier)  MsgIdentifier=8197  MsgLength=8  SignalInfo=VCU_AcmSt$38$2$1$2$1$0$1$0$0$3$#VCU_AcmTemp$24$8$1$2$1$0$1$-50$-50$200$#VCU_BmsSt$32$2$1$2$1$0$1$0$0$3$#VCU_BmsTemp$0$8$1$2$1$0$1$-50$-50$200$#VCU_DcdcSt$40$2$1$2$1$0$1$0$0$3$#VCU_McuSt$34$2$1$2$1$0$1$0$0$3$#VCU_McuTemp$8$8$1$2$1$0$1$-50$-50$200$#VCU_RcuSt$36$2$1$2$1$0$1$0$0$3$#VCU_RcuTemp$16$8$1$2$1$0$1$-50$-50$200$#  NSignals=9  StartBits=str2num('[int32(38);int32(24);int32(32);int32(0);int32(40);int32(34);int32(8);int32(36);int32(16)]')  SignalSizes=str2num('[int32(2);int32(8);int32(2);int32(8);int32(2);int32(2);int32(8);int32(2);int32(8)]')  ByteOrders=str2num('[int32(1);int32(1);int32(1);int32(1);int32(1);int32(1);int32(1);int32(1);int32(1)]')  DataTypes=str2num('[int32(2);int32(2);int32(2);int32(2);int32(2);int32(2);int32(2);int32(2);int32(2)]')  MultiplexTypes=str2num('[int32(1);int32(1);int32(1);int32(1);int32(1);int32(1);int32(1);int32(1);int32(1)]')  MultiplexValues=str2num('[double(0);double(0);double(0);double(0);double(0);double(0);double(0);double(0);double(0)]')  Factors=str2num('[double(1);double(1);double(1);double(1);double(1);double(1);double(1);double(1);double(1)]')  Offsets=str2num('[double(0);double(-50);double(0);double(-50);double(0);double(0);double(-50);double(0);double(-50)]')  Minimums=str2num('[double(0);double(-50);double(0);double(-50);double(0);double(0);double(-50);double(0);double(-50)]')  Maximums=str2num('[double(3);double(200);double(3);double(200);double(3);double(3);double(200);double(3);double(200)]')  Remote=off  ApplyMinMax=off  BusOutput=on
      settings: SourceProductName=Simulink Real-Time  SourceProductBaseCode=XP  DataFormat=CANdb specified signals
  wires:
  Bus Selector/2 -> FCAN_Send_ID_0x2001/2  "<Length>"
  Bus Selector/1 -> FCAN_Send_ID_0x2001/1  "<Data>"
  VCU2AUTO1/1 -> Bus Selector/1
  VCU2AUTO2/1 -> Bus Selector1/1
  Bus Selector1/1 -> FCAN_Send_ID_0x2002/1  "<Data>"
  Bus Selector1/2 -> FCAN_Send_ID_0x2002/2  "<Length>"
  Bus Selector2/2 -> FCAN_Send_ID_0x2003/2  "<Length>"
  Bus Selector2/1 -> FCAN_Send_ID_0x2003/1  "<Data>"
  VCU2AUTO3/1 -> Bus Selector2/1
  VCU2AUTO4/1 -> Bus Selector3/1
  Bus Selector3/1 -> FCAN_Send_ID_0x2004/1  "<Data>"
  Bus Selector3/2 -> FCAN_Send_ID_0x2004/2  "<Length>"
  Bus Selector4/2 -> FCAN_Send_ID_0x2005/2  "<Length>"
  Bus Selector4/1 -> FCAN_Send_ID_0x2005/1  "<Data>"
  VCU2AUTO5/1 -> Bus Selector4/1
  "CAN_INFO "/1 -> [CAN_INFO]
  [CAN_INFO] -> Bus Selector5/1
  Bus Selector5/1 -> Subsystem/1("Press "), Data Type Conversion/1  "<BDX_BrakePressure>"
  Bus Selector6/7 -> Data Type Conversion14/1  "<PwrTotal>"
  Bus Selector6/5 -> Data Type Conversion12/1  "<BMS_LineVoltage>"
  Bus Selector6/4 -> 1-D Lookup Table/1  "<APPSOC>"
  Bus Selector6/3 -> Data Type Conversion10/1  "<BMS_PackCurrent>"
  [CAN_INFO] -> Bus Selector6/1
  [CAN_INFO] -> Bus Selector7/1
  [CAN_INFO] -> Bus Selector8/1
  [CAN_INFO] -> Bus Selector12/1, Bus Selector11/1, Bus Selector10/1, Bus Selector9/1
  Bus Selector9/1 -> Data Type Conversion23/1  "<Work_STS_Comp>"
  Bus Selector6/1 -> Data Type Conversion8/1  "<BMS_SupplyVol>"
  Bus Selector9/4 -> Data Type Conversion25/1  "<BMS_BatteryState>"
  Bus Selector9/5 -> Data Type Conversion26/1  "<BMS_MaxBatteryTemp>"
  Bus Selector9/6 -> Data Type Conversion27/1  "<DCDC_WrkSts>"
  Bus Selector5/4 -> Data Type Conversion3/1  "<VehTrq>"
  Bus Selector5/6 -> Data Type Conversion5/1  "<ModeStr>"
  Bus Selector5/7 -> Data Type Conversion6/1  "<Ready>"
  Bus Selector5/8 -> Gain4/1  "<VehSpd>"
  Bus Selector5/2 -> Subsystem/2(fault)  "<BDX_BP_fault>"
  Subsystem/1(Out1) -> Data Type Conversion1/1
  Data Type Conversion/1 -> VCU2AUTO1/1
  Data Type Conversion1/1 -> VCU2AUTO1/2
  Data Type Conversion2/1 -> VCU2AUTO1/3
  Data Type Conversion3/1 -> VCU2AUTO1/4
  Data Type Conversion4/1 -> VCU2AUTO1/5
  Data Type Conversion5/1 -> VCU2AUTO1/6
  Data Type Conversion6/1 -> VCU2AUTO1/7
  Data Type Conversion7/1 -> VCU2AUTO1/8
  Bus Selector6/6 -> Divide/1  "<MCU_SpdEst>"
  Constant/1 -> Divide/2
  Divide/1 -> Data Type Conversion13/1
  Bus Selector7/1 -> Gain5/1  "<MCU_TrqEst>"
  Bus Selector7/2 -> Gain6/1  "<MCU_TrqEst>"
  Bus Selector7/3 -> Data Type Conversion17/1  "<MCU_TrqEst>"
  Bus Selector7/4 -> Gain8/1  "<MCU_TrqEst>"
  Constant2/1 -> Product6/2, Product7/2, Product5/2, Product4/2
  Bus Selector8/4 -> Product7/1  "<MCU_SpdEst>"
  Product7/1 -> Gain3/1
  Product6/1 -> Gain2/1
  Bus Selector8/3 -> Product6/1  "<MCU_SpdEst>"
  Bus Selector8/2 -> Product5/1  "<MCU_SpdEst>"
  Product5/1 -> Gain1/1
  Product4/1 -> Gain/1
  Bus Selector8/1 -> Product4/1  "<MCU_SpdEst>"
  Gain/1 -> Data Type Conversion19/1
  Gain1/1 -> Data Type Conversion20/1
  Gain2/1 -> Data Type Conversion21/1
  Gain3/1 -> Data Type Conversion22/1
  Data Type Conversion8/1 -> VCU2AUTO2/1
  Data Type Conversion9/1 -> VCU2AUTO2/2
  Data Type Conversion10/1 -> VCU2AUTO2/3
  Data Type Conversion11/1 -> VCU2AUTO2/4
  Data Type Conversion12/1 -> VCU2AUTO2/5
  Data Type Conversion13/1 -> VCU2AUTO2/6
  Data Type Conversion14/1 -> VCU2AUTO2/7
  Bus Selector6/2 -> Data Type Conversion9/1  "<LiqudLevel>"
  Bus Selector9/2 -> Max/1  "<BatTempOut>"
  Data Type Conversion15/1 -> VCU2AUTO3/1
  Data Type Conversion16/1 -> VCU2AUTO3/2
  Data Type Conversion17/1 -> VCU2AUTO3/3
  Data Type Conversion18/1 -> VCU2AUTO3/4
  Data Type Conversion19/1 -> VCU2AUTO4/1
  Data Type Conversion20/1 -> VCU2AUTO4/2
  Data Type Conversion21/1 -> VCU2AUTO4/3
  Data Type Conversion22/1 -> VCU2AUTO4/4
  Data Type Conversion23/1 -> VCU2AUTO5/1
  Data Type Conversion24/1 -> VCU2AUTO5/2
  Data Type Conversion25/1 -> VCU2AUTO5/3
  Data Type Conversion26/1 -> VCU2AUTO5/4
  Data Type Conversion27/1 -> VCU2AUTO5/5
  Bus Selector10/1 -> Max1/1  "<MCU_N_FaultGrade>"
  Bus Selector10/2 -> Max1/2  "<MCU_N_FaultGrade>"
  Bus Selector10/3 -> Max1/3  "<MCU_N_FaultGrade>"
  Bus Selector10/4 -> Max1/4  "<MCU_N_FaultGrade>"
  Bus Selector10/5 -> Max1/5  "<MCU_N_FaultGrade>"
  Max1/1 -> Saturation/1
  Data Type Conversion28/1 -> VCU2AUTO5/6
  Bus Selector12/1 -> Data Type Conversion29/1  "<RCU_ActWorkSts>"
  Bus Selector12/2 -> Max2/1  "<RCU_GCUISGMotorActTemp>"
  Bus Selector12/3 -> Max2/2  "<RCU_GCUISGInverterActTemp>"
  Max2/1 -> Saturation2/1
  Data Type Conversion29/1 -> VCU2AUTO5/8
  Data Type Conversion30/1 -> VCU2AUTO5/9
  Data Type Conversion31/1 -> VCU2AUTO5/7
  Max3/1 -> Saturation1/1
  Bus Selector11/1 -> Max3/1  "<MCU_nControllerTemp>"
  Bus Selector11/2 -> Max3/2  "<MCU_nMotorTemp>"
  Bus Selector11/3 -> Max3/3  "<MCU_nControllerTemp>"
  Bus Selector11/4 -> Max3/4  "<MCU_nMotorTemp>"
  Bus Selector11/5 -> Max3/5  "<MCU_nControllerTemp>"
  Bus Selector11/6 -> Max3/6  "<MCU_nMotorTemp>"
  Bus Selector11/7 -> Max3/7  "<MCU_nControllerTemp>"
  Bus Selector11/8 -> Max3/8  "<MCU_nMotorTemp>"
  Bus Selector11/9 -> Max3/9  "<MCU_nControllerTemp>"
  Bus Selector11/10 -> Max3/10  "<MCU_nMotorTemp>"
  Saturation/1 -> Data Type Conversion28/1
  Saturation1/1 -> Data Type Conversion31/1
  Saturation2/1 -> Data Type Conversion30/1
  Data Store Read/1 -> Data Type Conversion4/1
  1-D Lookup Table/1 -> Data Type Conversion11/1
  Bus Selector5/3 -> Terminator/1  "<ESM_BMSChargSts>"
  Bus Selector5/5 -> Terminator1/1  "<BDX_SteeringAngle>"
  Subsystem1/1(Out1) -> Data Type Conversion2/1
  Gain4/1 -> Data Type Conversion7/1
  Gain5/1 -> Data Type Conversion15/1
  Gain6/1 -> Data Type Conversion16/1
  Gain8/1 -> Data Type Conversion18/1
  Bus Selector9/3 -> Max/2  "<PTC_Coolanttemperature>"
  Max/1 -> Data Type Conversion24/1

== system VehCtrl20260630_18B/SigOut/BDX ==
  "BDX_OUT " : Inport
  Trigger : TriggerPort  VariantControl=Variant  PortDimensions=1
  Bus Selector : BusSelector  OutputSignals=Data,Length
  Bus Selector1 : BusSelector  OutputSignals=SuspDownValve,Pump,WidthShortenValve,WidthLengthenValve,SuspUpValve,EpbValve,SteerValveL,SteerValveR,BrkValve
  Bus Selector3 : BusSelector  OutputSignals=SuspDownValve,WidthShortenValve,WidthLengthenValve,SuspUpValve,SteerValveL,SteerValveR,BrkValve
  Constant1 : Constant  Value=8
  Constant2 : Constant  Value=hex2dec('40')
  Constant3 : Constant  Value=hex2dec('04')
  Constant4 : Constant  Value=hex2dec('10')
  Constant5 : Constant  Value=0
  Data Store Read : DataStoreRead  DataStoreName=DO_Y1
  Data Store Read1 : DataStoreRead  DataStoreName=DO_Y2
  Data Store Read2 : DataStoreRead  DataStoreName=DO_Y3
  Data Store Read3 : DataStoreRead  DataStoreName=DO_Y4
  Data Store Read4 : DataStoreRead  DataStoreName=DO_Y5
  Data Store Read5 : DataStoreRead  DataStoreName=DO_Y6
  Data Store Read6 : DataStoreRead  DataStoreName=DO_Z1
  Data Store Read7 : DataStoreRead  DataStoreName=DO_Z1
  Data Store Read8 : DataStoreRead  DataStoreName=DO_Y11
  Data Store Write : DataStoreWrite  DataStoreName=DO_Y11
  Data Type Conversion : DataTypeConversion
  Data Type Conversion1 : DataTypeConversion
  Data Type Conversion{2..5} (4 alike) : DataTypeConversion  OutDataTypeStr=boolean
  FCAN_Send_ID_0x3FF : mbd_mpc574x_ec_toolbox/Communication Blocks/CAN Blocks/FCAN_Send  Priority=2  can_instance=2  can_mode=Non-blocking  can_timeout_ms=0  can_mb_idx=45  can_extended_id=off  can_is_remote=off  can_id=130  show_adv_opts=off  can_fd_enable=off  can_enable_brs=off  can_fd_padding=0
      settings: SourceProductName=NXP Model-Based Design Toolbox for MPC57xx MCUs
  FCAN_Send_ID_0x3FF1 : mbd_mpc574x_ec_toolbox/Communication Blocks/CAN Blocks/FCAN_Send  Priority=2  can_instance=2  can_mode=Non-blocking  can_timeout_ms=0  can_mb_idx=51  can_extended_id=off  can_is_remote=off  can_id=605  show_adv_opts=off  can_fd_enable=off  can_enable_brs=off  can_fd_padding=0
      settings: SourceProductName=NXP Model-Based Design Toolbox for MPC57xx MCUs
  Logical Operator : Logic  Operator=OR  Inputs=8  AllPortsSameDT=off  OutDataTypeStr=boolean
  MCU_ : canmsglib/CAN Pack  CANdbFile=D:\VCU\VCU_AgriculturalMachinery_ChangChun\CAN协议8.4\液压\BDX_DBC_VCU_CAN0.dbc  MsgList=AVCU_130  MsgName=AVCU_130  MsgIDType=Standard (11-bit identifier)  MsgIdentifier=304  MsgLength=8  SignalInfo=DO_Y1$49$1$1$2$1$0$1$0$0$1$#DO_Y10$58$1$1$2$1$0$1$0$0$1$#DO_Y11$59$1$1$2$1$0$1$0$0$1$#DO_Y2$50$1$1$2$1$0$1$0$0$1$#DO_Y3$51$1$1$2$1$0$1$0$0$1$#DO_Y4$52$1$1$2$1$0$1$0$0$1$#DO_Y5$53$1$1$2$1$0$1$0$0$1$#DO_Y6$54$1$1$2$1$0$1$0$0$1$#DO_Y7$55$1$1$2$1$0$1$0$0$1$#DO_Y8$56$1$1$2$1$0$1$0$0$1$#DO_Y9$57$1$1$2$1$0$1$0$0$1$#DO_Z1$48$1$1$2$1$0$1$0$0$1$#PWM_S1$0$16$1$2$1$0$4.880000e-02$0$0$100$#PWM_S2$16$16$1$2$1$0$4.880000e-02$0$0$100$#PWM_S3$32$16$1$2$1$0$4.880000e-02$0$0$100$#  NSignals=15  StartBits=str2num('[int32(49);int32(58);int32(59);int32(50);int32(51);int32(52);int32(53);int32(54);int32(55);int32(56);int32(57);int32(48);int32(0);int32(16);int32(32)]')  SignalSizes=str2num('[int32(1);int32(1);int32(1);int32(1);int32(1);int32(1);int32(1);int32(1);int32(1);int32(1);int32(1);int32(1);int32(16);int32(16);int32(16)]')  ByteOrders=str2num('[int32(1);int32(1);int32(1);int32(1);int32(1);int32(1);int32(1);int32(1);int32(1);int32(1);int32(1);int32(1);int32(1);int32(1);int32(1)]')  DataTypes=str2num('[int32(2);int32(2);int32(2);int32(2);int32(2);int32(2);int32(2);int32(2);int32(2);int32(2);int32(2);int32(2);int32(2);int32(2);int32(2)]')  MultiplexTypes=str2num('[int32(1);int32(1);int32(1);int32(1);int32(1);int32(1);int32(1);int32(1);int32(1);int32(1);int32(1);int32(1);int32(1);int32(1);int32(1)]')  MultiplexValues=str2num('[double(0);double(0);double(0);double(0);double(0);double(0);double(0);double(0);double(0);double(0);double(0);double(0);double(0);double(0);double(0)]')  Factors=str2num('[double(1);double(1);double(1);double(1);double(1);double(1);double(1);double(1);double(1);double(1);double(1);double(1);double(4.880000e-02);double(4.880000e-02);double(4.880000e-02)]')  Offsets=str2num('[double(0);double(0);double(0);double(0);double(0);double(0);double(0);double(0);double(0);double(0);double(0);double(0);double(0);double(0);double(0)]')  Minimums=str2num('[double(0);double(0);double(0);double(0);double(0);double(0);double(0);double(0);double(0);double(0);double(0);double(0);double(0);double(0);double(0)]')  Maximums=str2num('[double(1);double(1);double(1);double(1);double(1);double(1);double(1);double(1);double(1);double(1);double(1);double(1);double(100);double(100);double(100)]')  Remote=off  ApplyMinMax=off  BusOutput=on
      settings: SourceProductName=Simulink Real-Time  SourceProductBaseCode=XP  DataFormat=CANdb specified signals
  Mux : Mux  Inputs=8
  Terminator : Terminator
  Terminator1 : Terminator
  wires:
  Bus Selector/2 -> FCAN_Send_ID_0x3FF/2  "<Length>"
  Bus Selector/1 -> FCAN_Send_ID_0x3FF/1  "<Data>"
  "BDX_OUT "/1 -> Bus Selector3/1, Bus Selector1/1
  MCU_/1 -> Bus Selector/1
  Data Store Read/1 -> MCU_/1
  Data Store Read1/1 -> MCU_/4
  Data Store Read2/1 -> MCU_/5
  Data Store Read3/1 -> MCU_/6
  Data Store Read4/1 -> MCU_/7
  Data Store Read5/1 -> MCU_/8
  Bus Selector1/5 -> MCU_/11  "<SuspUpValve>"
  Bus Selector1/4 -> MCU_/10  "<WidthLengthenValve>"
  Bus Selector1/1 -> MCU_/2  "<SuspDownValve>"
  Bus Selector1/3 -> MCU_/9  "<WidthShortenValve>"
  Bus Selector1/6 -> Terminator/1  "<EpbValve>"
  Bus Selector1/7 -> MCU_/13  "<SteerValveL>"
  Bus Selector1/9 -> MCU_/15  "<BrkValve>"
  Bus Selector1/8 -> MCU_/14  "<SteerValveR>"
  Data Store Read6/1 -> MCU_/12
  Data Store Read8/1 -> MCU_/3
  Bus Selector1/2 -> Terminator1/1  "<Pump>"
  Bus Selector3/6 -> Data Type Conversion2/1  "<SteerValveR>"
  Bus Selector3/7 -> Data Type Conversion3/1  "<BrkValve>"
  Bus Selector3/5 -> Data Type Conversion4/1  "<SteerValveL>"
  Data Type Conversion4/1 -> Logical Operator/6
  Data Type Conversion2/1 -> Logical Operator/7
  Data Type Conversion3/1 -> Logical Operator/8
  Bus Selector3/4 -> Logical Operator/5  "<SuspUpValve>"
  Bus Selector3/3 -> Logical Operator/4  "<WidthLengthenValve>"
  Bus Selector3/2 -> Logical Operator/3  "<WidthShortenValve>"
  Bus Selector3/1 -> Logical Operator/2  "<SuspDownValve>"
  Data Store Read7/1 -> Logical Operator/1
  Logical Operator/1 -> Data Type Conversion5/1
  Data Type Conversion5/1 -> Data Store Write/1
  Constant4/1 -> Mux/3
  Constant3/1 -> Mux/2
  Mux/1 -> Data Type Conversion/1
  Constant1/1 -> Data Type Conversion1/1
  Data Type Conversion1/1 -> FCAN_Send_ID_0x3FF1/2
  Constant5/1 -> Mux/5, Mux/6, Mux/8, Mux/7, Mux/4
  Data Type Conversion/1 -> FCAN_Send_ID_0x3FF1/1
  Constant2/1 -> Mux/1

== system VehCtrl20260630_18B/SigOut/BMS ==
  "BMS_OUT " : Inport
  Trigger : TriggerPort  VariantControl=Variant  PortDimensions=1
  Bus Selector1 : BusSelector  OutputSignals=VCU_Maincircuitcommand
  Constant : Constant  Value=0  OutDataTypeStr=uint8
  Constant1 : Constant  Value=8  OutDataTypeStr=uint8
  Data Type Conversion : DataTypeConversion  OutDataTypeStr=uint8
  FCAN_Send_ID_0x3FF1 : mbd_mpc574x_ec_toolbox/Communication Blocks/CAN Blocks/FCAN_Send  Priority=2  can_instance=2  can_mode=Non-blocking  can_timeout_ms=0  can_mb_idx=43  can_extended_id=on  can_is_remote=off  can_id=0C014785  show_adv_opts=off  can_fd_enable=off  can_enable_brs=off  can_fd_padding=0
      settings: SourceProductName=NXP Model-Based Design Toolbox for MPC57xx MCUs
  Gain : Gain  Gain=4  OutDataTypeStr=uint8
  Mux : Mux  Inputs=8
  VCU2MCU1_2 : canmsglib/CAN Pack  Commented=on  CANdbFile=D:\VCU\VCU_AgriculturalMachinery_ChangChun\CAN协议8.4\BMS\BMS_DBC_Sheet1.dbc  MsgList=(none)  MsgName=VCUtoBMS  MsgIDType=Extended (29-bit identifier)  MsgIdentifier=201410437  MsgLength=8  SignalInfo=VCU_Maincircuitcommand$2$2$1$2$1$0$1$0$0$3$#  NSignals=1  StartBits=str2num('[int32(2)]')  SignalSizes=str2num('[int32(2)]')  ByteOrders=str2num('[int32(1)]')  DataTypes=str2num('[int32(2)]')  MultiplexTypes=str2num('[int32(1)]')  MultiplexValues=str2num('[double(0)]')  Factors=str2num('[double(1)]')  Offsets=str2num('[double(0)]')  Minimums=str2num('[double(0)]')  Maximums=str2num('[double(3)]')  Remote=off  ApplyMinMax=off  BusOutput=on
      settings: SourceProductName=Simulink Real-Time  SourceProductBaseCode=XP  DataFormat=manually specified signals
  wires:
  "BMS_OUT "/1 -> Bus Selector1/1
  Constant1/1 -> FCAN_Send_ID_0x3FF1/2
  Bus Selector1/1 -> Gain/1  "<VCU_Maincircuitcommand>"
  Gain/1 -> Data Type Conversion/1
  Constant/1 -> Mux/3, Mux/6, Mux/7, Mux/8, Mux/5, Mux/4, Mux/2
  Data Type Conversion/1 -> Mux/1
  Mux/1 -> FCAN_Send_ID_0x3FF1/1

== system VehCtrl20260630_18B/SigOut/DCDC ==
  "DCDC_OUT " : Inport
  Trigger : TriggerPort  VariantControl=Variant  PortDimensions=1
  Bus Selector : BusSelector  OutputSignals=Data,Length
  Bus Selector1 : BusSelector  OutputSignals=DCDC_Enable
  Constant : Constant  Value=0
  Data Type Conversion : DataTypeConversion
  FCAN_Send_ID_0x3FF : mbd_mpc574x_ec_toolbox/Communication Blocks/CAN Blocks/FCAN_Send  Priority=2  can_instance=1  can_mode=Non-blocking  can_timeout_ms=0  can_mb_idx=44  can_extended_id=on  can_is_remote=off  can_id=10262B27  show_adv_opts=off  can_fd_enable=off  can_enable_brs=off  can_fd_padding=0
      settings: SourceProductName=NXP Model-Based Design Toolbox for MPC57xx MCUs
  VCU2MCU1_1 : canmsglib/CAN Pack  CANdbFile=D:\VCU\VCU_AgriculturalMachinery_ChangChun\CAN协议8.4\DCDC\DCDC_DBC_VCU_CAN0.dbc  MsgList=DCDC_Cmd1  MsgName=DCDC_Cmd1  MsgIDType=Extended (29-bit identifier)  MsgIdentifier=270936871  MsgLength=8  SignalInfo=DCDC_Ctrwrkcmd$0$2$1$2$1$0$1$0$0$3$#DCDC_Rstwrkcmd$56$2$1$2$1$0$1$0$0$3$#  NSignals=2  StartBits=str2num('[int32(0);int32(56)]')  SignalSizes=str2num('[int32(2);int32(2)]')  ByteOrders=str2num('[int32(1);int32(1)]')  DataTypes=str2num('[int32(2);int32(2)]')  MultiplexTypes=str2num('[int32(1);int32(1)]')  MultiplexValues=str2num('[double(0);double(0)]')  Factors=str2num('[double(1);double(1)]')  Offsets=str2num('[double(0);double(0)]')  Minimums=str2num('[double(0);double(0)]')  Maximums=str2num('[double(3);double(3)]')  Remote=off  ApplyMinMax=off  BusOutput=on
      settings: SourceProductName=Simulink Real-Time  SourceProductBaseCode=XP  DataFormat=CANdb specified signals
  wires:
  Bus Selector/2 -> FCAN_Send_ID_0x3FF/2  "<Length>"
  Bus Selector/1 -> FCAN_Send_ID_0x3FF/1  "<Data>"
  "DCDC_OUT "/1 -> Bus Selector1/1
  VCU2MCU1_1/1 -> Bus Selector/1
  Bus Selector1/1 -> VCU2MCU1_1/1  "<DCDC_Enable>"
  Data Type Conversion/1 -> VCU2MCU1_1/2
  Constant/1 -> Data Type Conversion/1

== system VehCtrl20260630_18B/SigOut/GPIO  ==
  note: LS
  note: PWM
  note: HS
  ETC : Subsystem
  HS : Subsystem
  PWM_OUT : Subsystem  Commented=on
  SPI0: LS09_14_15_16_1_2_11_4 : Subsystem
  SPI3: LS03_06_07_08_10_12_13_17_18_19 : Subsystem
